simulink model "model_math_loc"  (R2019a)
settings: Solver=FixedStepAuto  StartTime=0.0  StopTime=10  FixedStep=0.01  RelTol=1e-3
undefined symbols (not defined in the file): K
settings Model: Creator=chute  LastModifiedBy=chute
settings DataIOCC: ReturnWorkspaceOutputs=off

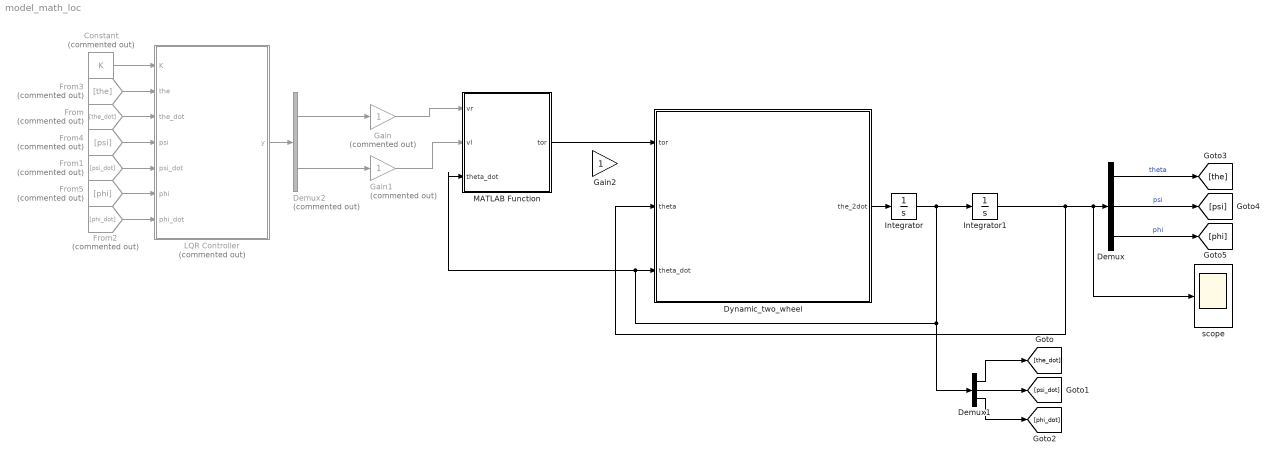
== system model_math_loc ==
  Constant : Constant  Commented=on  Value=K
  Demux : Demux  Outputs=3
  Demux1 : Demux  Outputs=3
  Demux2 : Demux  Commented=on  Outputs=2
  Dynamic_two_wheel : MATLAB Function  TreatAsAtomicUnit=on
  From : From  Commented=on  GotoTag=the_dot
  From1 : From  Commented=on  GotoTag=psi_dot
  From2 : From  Commented=on  GotoTag=phi_dot
  From3 : From  Commented=on  GotoTag=the
  From4 : From  Commented=on  GotoTag=psi
  From5 : From  Commented=on  GotoTag=phi
  Gain : Gain  Commented=on
  Gain1 : Gain  Commented=on
  Gain2 : Gain
  Integrator : Integrator  InitialCondition=[0.01;0.01;0.01]
  Integrator1 : Integrator  InitialCondition=[0.01;0.01;0.3]
  "LQR Controller " : MATLAB Function  Commented=on  TreatAsAtomicUnit=on
  MATLAB Function : MATLAB Function  TreatAsAtomicUnit=on
  scope : Scope
  wires:
  Demux2/1 -> Gain/1
  Dynamic_two_wheel/1(the_2dot) -> Integrator/1
  Integrator/1 -> Integrator1/1, MATLAB Function/3(theta_dot), Dynamic_two_wheel/3(theta_dot), Demux1/1
  Integrator1/1 -> Dynamic_two_wheel/2(theta), scope/1, Demux/1
  "LQR Controller "/1(y) -> Demux2/1
  Demux1/1 -> [the_dot]
  Demux1/2 -> [psi_dot]
  Demux1/3 -> [phi_dot]
  From/1 -> "LQR Controller "/3(the_dot)
  From1/1 -> "LQR Controller "/5(psi_dot)
  From2/1 -> "LQR Controller "/7(phi_dot)
  Demux/3 -> [phi]  "phi"
  Demux/2 -> [psi]  "psi"
  Demux/1 -> [the]  "theta"
  From3/1 -> "LQR Controller "/2(the)
  From5/1 -> "LQR Controller "/6(phi)
  From4/1 -> "LQR Controller "/4(psi)
  Constant/1 -> "LQR Controller "/1(K)
  Demux2/2 -> Gain1/1
  Gain/1 -> MATLAB Function/1(vr)
  Gain1/1 -> MATLAB Function/2(vl)
  MATLAB Function/1(tor) -> Dynamic_two_wheel/1(tor)

== matlab function model_math_loc/Dynamic_two_wheel ==
  data: tor input; the_2dot output; theta input; theta_dot input
function the_2dot = fcn(tor,theta,theta_dot)
%% declare the parameter
g =s9.81; % gravity acceleration
m =0.046; % wheel weight
R =0.3375; % Wheel radius
M =0.95;  % body weight
W =0.22; % Body width
D =0.1; % Body depth
H =0.121;% Body Height
L =0.144/2;% distance
J_psi  = M*L^2/3; % Body inertia moment
Jw = m*R^2/2;  %Wheel inertia moment
J_phi = M*(W^2+D^2)/12; % Body yaw inertia moment
Jm = 0.00001; % Dc motor inertia moment
% Rm = 8.6123; % Dc motor resitance
% Kb = 0.225; % DC motor EMF
% Kt = 3.0896; % DC motor torque const
% fm = 0.0022; % friction cof between body and DC motor.
% fw = 0; % friction cof between wheel and floor



n =30 ; %gear ratio
% anp = n*Kt/Rm;
% bet = n*Kt*Kb/Rm +fm;

% the = theta(1);
% psi = theta(2);
% phi = theta(3);

the_dot = theta_dot(1);
psi_dot = theta_dot(2);
phi_dot = theta_dot(3);

the = theta(1);
psi = theta(2);
phi = theta(3);


M1 = ...
[2*Jw + 2*Jm*n^2 + R^2*(M + 2*m),L*M*R*cos(psi) - 2*Jm*n^2,0;
 L*M*R*cos(psi) - 2*Jm*n^2,J_psi + L^2*M + 2*Jm*n^2,0;
 0,0,J_phi + (W^2*m)/2 + L^2*M*sin(psi)^2 + (W^2*(Jw + Jm*n^2))/(2*R^2)];


C = ...
[0,-L*M*R*psi_dot*sin(psi),0;
 0,0,-L^2*M*phi_dot*cos(psi)*sin(psi);
 0,L^2*M*phi_dot*cos(psi)*sin(psi),L^2*M*psi_dot*cos(psi)*sin(psi)];

G=...
[0;
-L*M*g*sin(psi);
0];
dei = transpose([the_dot  psi_dot  phi_dot]);

the_2dot = inv(M1)*(tor-C*dei-G-5*theta_dot);

== matlab function model_math_loc/MATLAB Function ==
  data: vr input; tor output; vl input; theta_dot input
function tor = fcn(vr,vl,theta_dot)
the_dot=theta_dot(1,1);
psi_dot=theta_dot(2,1);
phi_dot=theta_dot(2,1);
g =9.81; % gravity acceleration
m =0.046; % wheel weight
R =0.3375; % Wheel radius
M =0.95;  % body weight
W =0.22; % Body width
D =0.1; % Body depth
H =0.121;% Body Height
L =0.144/2;% distance
J_psi  = M*L^2/3; % Body inertia moment
Jw = m*R^2/2;  %Wheel inertia moment
J_phi = M*(W^2+D^2)/12; % Body yaw inertia moment
Jm = 0.00001; % Dc motor inertia moment
Rm = 8.6123; % Dc motor resitance
Kb = 0.225; % DC motor EMF
Kt = 3.0896; % DC motor torque const
fm = 0.0022; % friction cof between body and DC motor.
fw = 0; % friction cof between wheel and floor
n =30 ; %gear ratio
anp = n*Kt/Rm;
bet = n*Kt*Kb/Rm +fm;
F_the = anp*(vl+vr)-2*(bet+fw)*the_dot+2*bet*psi_dot;
F_psi = -anp*(vl+vr)+2*bet*the_dot-2*bet*psi_dot;
F_phi = W*anp*(vr-vl)/(2*R)-W^2*((bet+fw)*phi_dot)/2*R^2;
tor =[F_the;F_psi;F_phi];
end

== matlab function model_math_loc/LQR Controller  ==
  data: K input; y output; the input; the_dot input; psi input; psi_dot input; phi input; phi_dot input
function y = fcn(K,the, the_dot, psi,psi_dot, phi, phi_dot)
XXX = [the;the_dot; psi;psi_dot; phi; phi_dot];
y = -K*XXX;
